simulink library "TorqueCommand"  (R2024a)
settings: Solver=VariableStepAuto  StartTime=0.0  StopTime=10.0  RelTol=1e-3
values from neighbouring files (symbols this model uses):
  RegenEnable : value not decoded    [TorqueCommand.sldd]
  TCEnable : value not decoded    [TorqueCommand.sldd]
undefined symbols (not defined in the file or in its folder): raptor_xcp_function
libraries: Raptor_lib x37, Utilities x7, simulink x6, slpidlib x1
settings Model: Creator=serga  LastModifiedBy=hyuga
settings ConfigComp: CovBoundaryAbsTol=1.0e-5

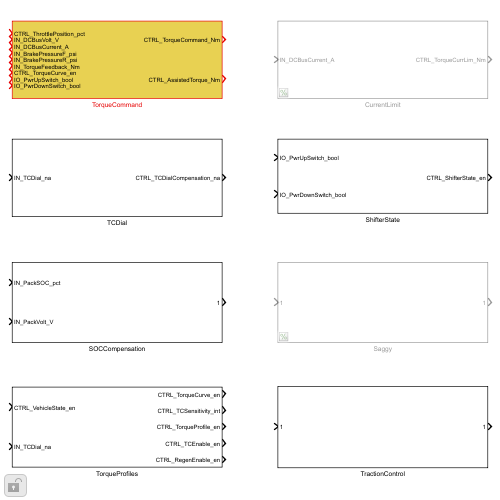
[thumbnail: Simulink's stored preview of the top-level diagram]
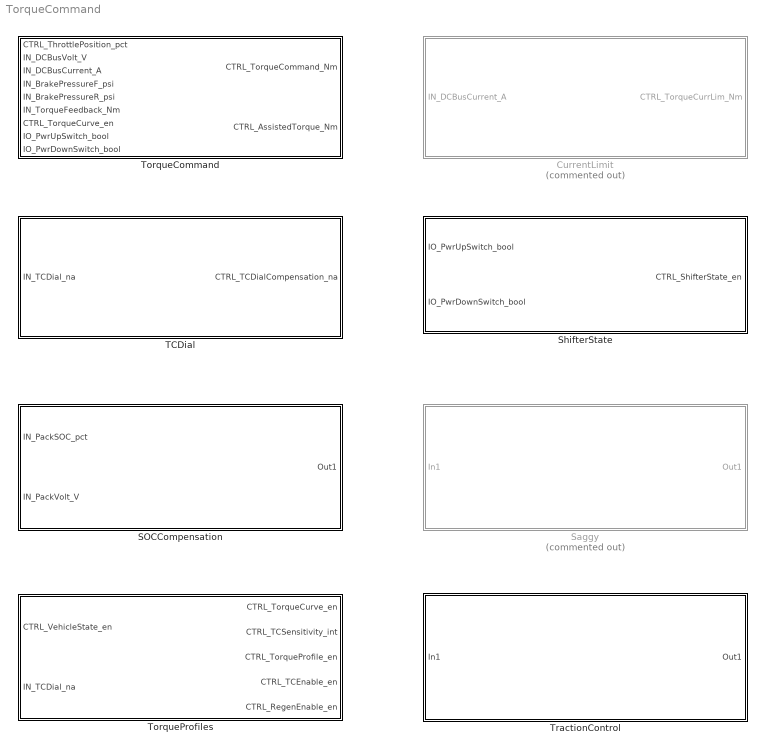
== system TorqueCommand ==
  CurrentLimit : Subsystem  Commented=on
  SOCCompensation : Subsystem
  Saggy : Subsystem  Commented=on
  ShifterState : Subsystem
  TCDial : Subsystem
  TorqueCommand : Subsystem
  TorqueProfiles : Subsystem
  TractionControl : Subsystem

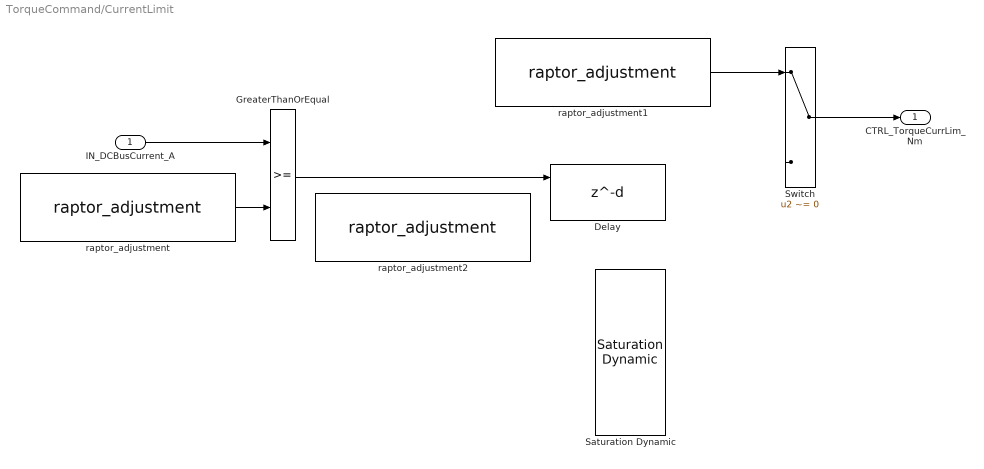
== system TorqueCommand/CurrentLimit ==
  IN_DCBusCurrent_A : Inport
  Delay : Delay  DelayLengthSource=Input port
      settings: InputPortMap=u0,p1
  GreaterThanOrEqual : RelationalOperator  OutDataTypeStr=boolean  RndMeth=Simplest  InputSameDT=off
  Saturation Dynamic : simulink/Discontinuities/Saturation Dynamic  OutMin=[]  OutMax=[]  OutDataTypeStr=Inherit: Same as second input  OutDataType=fixdt(1, 16)  OutScaling=2^-10  DoSatur=off
  Switch : Switch  Criteria=u2 ~= 0  SaturateOnIntegerOverflow=off  InputSameDT=off
  raptor_adjustment : Raptor_lib/Data Storage/raptor_adjustment  paramName='CTRL_DCBusOverCurrThresh_A'  nameSource=Parameter  initValue=125  dataType=uint8  storage=Calibration  calDispType=Number  calEnum={'False', 'True'}  calGain=1.0  calOffset=0.0  calMax=inf  calMin=-inf  calFormat='-1'  calUnit=''  calHelp=''  calAccess=1  calFunction=raptor_xcp_function(gcb)  calDispHeaders=off  calColHeaders={'Col1' 'Col2' 'Col3'}  calRowHeaders={'Row1' 'Row2' 'Row3'}
      settings: SourceProductName=Raptor
  raptor_adjustment1 : Raptor_lib/Data Storage/raptor_adjustment  paramName='CTRL_TorqueCurrLim_Nm'  nameSource=Parameter  initValue=100  dataType=double  storage=Calibration  calDispType=Number  calEnum={'False', 'True'}  calGain=1.0  calOffset=0.0  calMax=inf  calMin=-inf  calFormat='-1'  calUnit=''  calHelp=''  calAccess=1  calFunction=raptor_xcp_function(gcb)  calDispHeaders=off  calColHeaders={'Col1' 'Col2' 'Col3'}  calRowHeaders={'Row1' 'Row2' 'Row3'}
      settings: SourceProductName=Raptor
  raptor_adjustment2 : Raptor_lib/Data Storage/raptor_adjustment  paramName='CTRL_TorqueCurrLim_Nm'  nameSource=Parameter  initValue=100  dataType=double  storage=Calibration  calDispType=Number  calEnum={'False', 'True'}  calGain=1.0  calOffset=0.0  calMax=inf  calMin=-inf  calFormat='-1'  calUnit=''  calHelp=''  calAccess=1  calFunction=raptor_xcp_function(gcb)  calDispHeaders=off  calColHeaders={'Col1' 'Col2' 'Col3'}  calRowHeaders={'Row1' 'Row2' 'Row3'}
      settings: SourceProductName=Raptor
  CTRL_TorqueCurrLim_Nm : Outport
  wires:
  IN_DCBusCurrent_A/1 -> GreaterThanOrEqual/1
  raptor_adjustment/1 -> GreaterThanOrEqual/2
  GreaterThanOrEqual/1 -> Delay/1
  Switch/1 -> CTRL_TorqueCurrLim_Nm/1
  raptor_adjustment1/1 -> Switch/1

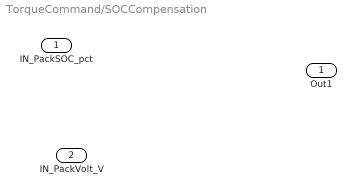
== system TorqueCommand/SOCCompensation ==
  IN_PackSOC_pct : Inport
  IN_PackVolt_V : Inport  Port=2
  Out1 : Outport

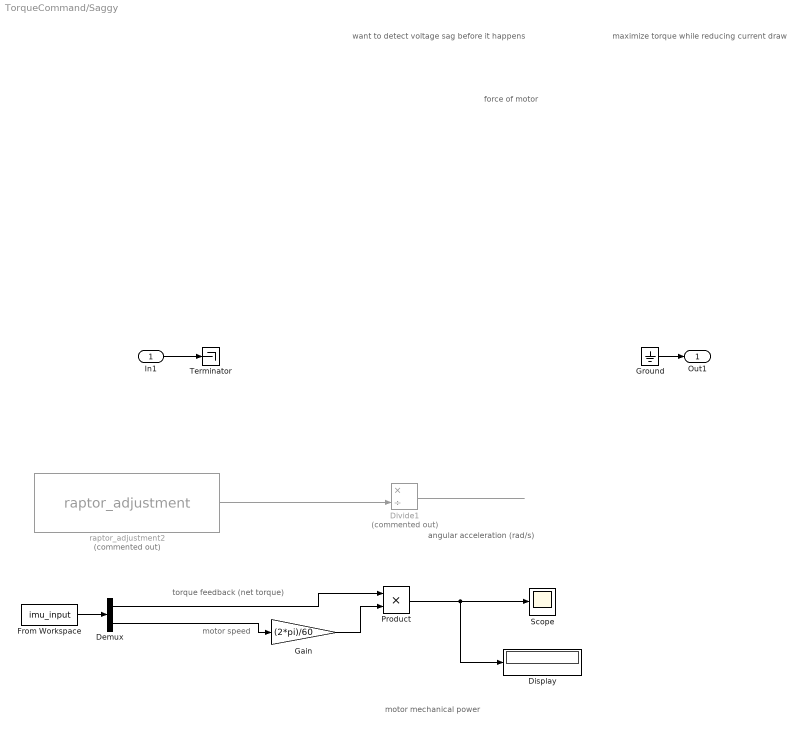
== system TorqueCommand/Saggy ==
  note: motor speed
  note: angular acceleration (rad/s)
  note: torque feedback (net torque)
  note: force of motor
  note: want to detect voltage sag before it happens
  note: maximize torque while reducing current draw
  note: motor mechanical power
  In1 : Inport
  Demux : Demux  Outputs=2
  Display : Display
  Divide1 : Product  Commented=on  Inputs=*/
  From Workspace : FromWorkspace  VariableName=imu_input  SampleTime=-1
  Gain : Gain  Gain=(2*pi)/60
  Ground : Ground
  Product : Product
  Scope : Scope
  Terminator : Terminator
  raptor_adjustment2 : Raptor_lib/Data Storage/raptor_adjustment  Commented=on  paramName='CTRL_MotorIntertia_kgm2'  nameSource=Parameter  initValue=0.0383  dataType=double  storage=Calibration  calDispType=Number  calEnum={'False', 'True'}  calGain=1.0  calOffset=0.0  calMax=inf  calMin=-inf  calFormat='-1'  calUnit=''  calHelp=''  calAccess=1  calFunction=raptor_xcp_function(gcb)  calDispHeaders=off  calColHeaders={'Col1' 'Col2' 'Col3'}  calRowHeaders={'Row1' 'Row2' 'Row3'}
      settings: SourceProductName=Raptor
  Out1 : Outport
  wires:
  In1/1 -> Terminator/1
  Ground/1 -> Out1/1
  raptor_adjustment2/1 -> Divide1/2
  Divide1/1 -> ?
  Gain/1 -> Product/2
  From Workspace/1 -> Demux/1
  Demux/1 -> Product/1
  Demux/2 -> Gain/1
  Product/1 -> Display/1, Scope/1

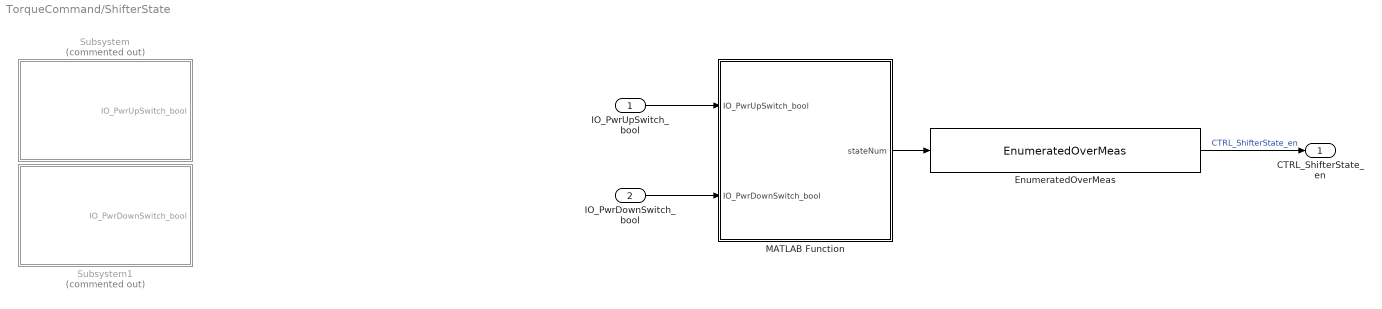
== system TorqueCommand/ShifterState ==
  IO_PwrUpSwitch_bool : Inport
  IO_PwrDownSwitch_bool : Inport  Port=2
  EnumeratedOverMeas : Utilities/EnumeratedOverMeas  sigName='CTRL_ShifterState_en'  enumName='TorqueState'
  MATLAB Function : MATLAB Function  TreatAsAtomicUnit=on
  Subsystem : Subsystem  Commented=on
  Subsystem1 : Subsystem  Commented=on
  CTRL_ShifterState_en : Outport
  wires:
  EnumeratedOverMeas/1 -> CTRL_ShifterState_en/1  "CTRL_ShifterState_en"
  MATLAB Function/1(stateNum) -> EnumeratedOverMeas/1
  IO_PwrDownSwitch_bool/1 -> MATLAB Function/2(IO_PwrDownSwitch_bool)
  IO_PwrUpSwitch_bool/1 -> MATLAB Function/1(IO_PwrUpSwitch_bool)

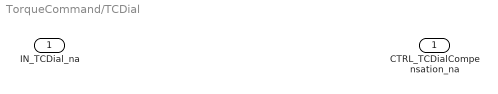
== system TorqueCommand/TCDial ==
  IN_TCDial_na : Inport
  CTRL_TCDialCompensation_na : Outport

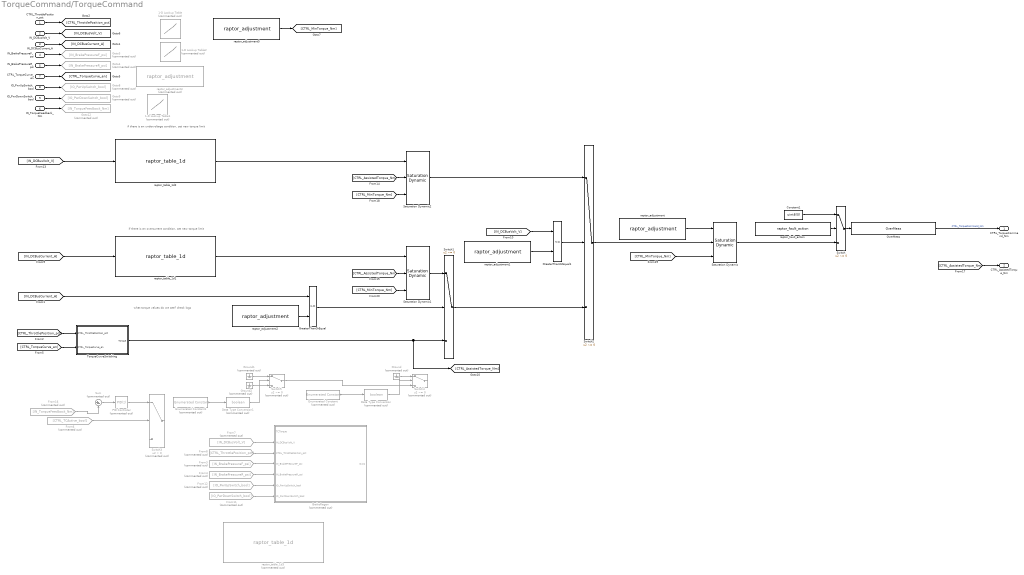
== system TorqueCommand/TorqueCommand ==
  note: if there is an undervoltage condition, set new torque limit
  note: what torque values do we see? check logs
  note: if there is an overcurrent condition, set new torque limit
  CTRL_ThrottlePosition_pct : Inport
  IN_DCBusVolt_V : Inport  Port=2
  IN_DCBusCurrent_A : Inport  Port=3
  IN_BrakePressureF_psi : Inport  Port=4
  IN_BrakePressureR_psi : Inport  Port=5
  IN_TorqueFeedback_Nm : Inport  Port=6
  CTRL_TorqueCurve_en : Inport  Port=7
  IO_PwrUpSwitch_bool : Inport  Port=8
  IO_PwrDownSwitch_bool : Inport  Port=9
  1-D Lookup Table : Lookup_n-D  Commented=on  NumberOfTableDimensions=1  BreakpointsForDimension1=[0;50;100;120;130;140;150;160;170;180;190;200;205;210;215;220;225;230;235;240;245;250;255;260;265;270;275;280;285;290;295;300]  Table=[200;200;200;200;200;200;200;200;200;200;200;200;200;200;200;200;200;200;200;200;200;200;195;190;185;180;175;170;165;160;155;150]  InternalRulePriority=Speed  RndMeth=Simplest
  1-D Lookup Table1 : Lookup_n-D  Commented=on  NumberOfTableDimensions=1  BreakpointsForDimension1=[0;5;10;15;20;25;30;35;40;45;50;55;60;65;70;75;80;85;90;95;100]  Table=[0;3;6;9;12;15;25;35;45;55;65;75;85;95;105;115;135;155;175;195;200]  InternalRulePriority=Speed  RndMeth=Simplest
  1-D Lookup Table2 : Lookup_n-D  Commented=on  NumberOfTableDimensions=1  BreakpointsForDimension1=[0;100;200;205;210;215;220;225;230;235;240;245;250;255;260;265;270;275;280;285;290;300;310;320;330;400]  Table=[0;0;0;25;50;100;125;150;155;160;165;170;175;180;185;190;192;194;196;198;200;200;200;200;200;200]  InternalRulePriority=Speed  RndMeth=Simplest
  BrakeRegen : Subsystem  Commented=on
  Constant1 : Constant  Value=uint8(0)
  Data Type Conversion : DataTypeConversion  Commented=on  OutDataTypeStr=boolean  SaturateOnIntegerOverflow=off  RndMeth=Floor
  Data Type Conversion1 : DataTypeConversion  Commented=on  OutDataTypeStr=boolean  SaturateOnIntegerOverflow=off  RndMeth=Floor
  Enumerated Constant : simulink/Sources/Enumerated Constant  Commented=on  OutDataTypeStr=Enum: RegenEnable  Value=RegenEnable.On  SampleTime=inf
  Enumerated Constant1 : simulink/Sources/Enumerated Constant  Commented=on  OutDataTypeStr=Enum: TCEnable  Value=TCEnable.On  SampleTime=inf
  From11 : From  Commented=on  GotoTag=IO_PwrDownSwitch_bool
  From12 : From  Commented=on  GotoTag=IO_PwrUpSwitch_bool
  From16 : From  Commented=on  GotoTag=IN_TorqueFeedback_Nm
  From3 : From  Commented=on  GotoTag=IN_BrakePressureF_psi
  From4 : From  Commented=on  GotoTag=IN_BrakePressureR_psi
  From6 : From  Commented=on  GotoTag=CTRL_TCActive_bool
  From7 : From  Commented=on  GotoTag=IN_DCBusVolt_V
  From8 : From  Commented=on  GotoTag=CTRL_ThrottlePosition_pct
  Goto12 : Goto  Commented=on  GotoTag=IN_TorqueFeedback_Nm
  Goto3 : Goto  Commented=on  GotoTag=IN_BrakePressureF_psi
  Goto4 : Goto  Commented=on  GotoTag=IN_BrakePressureR_psi
  Goto8 : Goto  Commented=on  GotoTag=IO_PwrUpSwitch_bool
  Goto9 : Goto  Commented=on  GotoTag=IO_PwrDownSwitch_bool
  GreaterThanOrEqual : RelationalOperator  OutDataTypeStr=boolean  RndMeth=Simplest  InputSameDT=off
  GreaterThanOrEqual1 : RelationalOperator  Operator=<=  OutDataTypeStr=boolean  RndMeth=Simplest  InputSameDT=off
  Ground : Ground  Commented=on
  Ground1 : Ground  Commented=on
  Ground2 : Ground  Commented=on
  OverMeas : Utilities/OverMeas  sigName='CTRL_TorqueCommand_Nm'  minimum=0  maximum=240
  PID Controller : slpidlib/PID Controller  Commented=on  Controller=PID  Form=Parallel  TimeDomain=Discrete-time  UseExternalTs=off  SampleTime=-1  IntegratorMethod=Forward Euler  FilterMethod=Forward Euler  ControllerParametersSource=internal  P=1  I=1  UseKiTs=off  D=0  UseExternalDerivativeSource=off  N=100  UseFilter=on  TunerSelectOption=Transfer Function Based (PID Tuner App)  InitialConditionSource=internal  InitialConditionForIntegrator=0  InitialConditionForFilter=0  DifferentiatorICPrevScaledInput=0  ExternalReset=none  TrackingMode=off  Kt=1  LimitOutput=off  SatLimitsSource=internal  UpperSaturationLimit=inf  LowerSaturationLimit=-inf  LinearizeAsGain=on  AntiWindupMode=none  Kb=1  LimitIntegrator=off  UpperIntegratorSaturationLimit=inf  LowerIntegratorSaturationLimit=-inf  POutMin=[]  POutMax=[]  IOutMin=[]  IOutMax=[]  DOutMin=[]  DOutMax=[]  NOutMin=[]  NOutMax=[]  SumOutMin=[]  SumOutMax=[]  SaturationOutMin=[]  SaturationOutMax=[]  PParamMin=[]  PParamMax=[]  IParamMin=[]  IParamMax=[]  DParamMin=[]  DParamMax=[]  NParamMin=[]  NParamMax=[]  KbParamMin=[]  KbParamMax=[]  KtParamMin=[]  KtParamMax=[]  KbOutMin=[]  KbOutMax=[]  KtOutMin=[]  KtOutMax=[]  IntegratorOutMin=[]  IntegratorOutMax=[]  FilterOutMin=[]  FilterOutMax=[]  SumI1OutMin=[]  SumI1OutMax=[]  SumI2OutMin=[]  SumI2OutMax=[]  SumI3OutMin=[]  SumI3OutMax=[]  SumI4OutMin=[]  SumI4OutMax=[]  SumDOutMin=[]  SumDOutMax=[]  DifferentiatorOutMin=[]  DifferentiatorOutMax=[]  FilterDiffOutCoefMin=[]  FilterDiffOutCoefMax=[]  ReciprocalOutMin=[]  ReciprocalOutMax=[]  SumDenOutMin=[]  SumDenOutMax=[]  SumNumOutMin=[]  SumNumOutMax=[]  DivideOutMin=[]  DivideOutMax=[]  UdiffTsProdOutMin=[]  UdiffTsProdOutMax=[]  NTsProdOutMin=[]  NTsProdOutMax=[]  UintegralTsProdOutMin=[]  UintegralTsProdOutMax=[]  UngainTsProdOutMin=[]  UngainTsProdOutMax=[]  ClampingZeroOutDataTypeStr=Inherit: Inherit via back propagation  ClampingZeroOutMin=[]  ClampingZeroOutMax=[]  FilterDenConstantOutDataTypeStr=Inherit: Inherit via back propagation  FilterDenConstantOutMin=[]  FilterDenConstantOutMax=[]  PCopyOutDataTypeStr=Inherit: Inherit via back propagation  PCopyOutMin=[]  PCopyOutMax=[]  NCopyOutDataTypeStr=Inherit: Inherit via back propagation  NCopyOutMin=[]  NCopyOutMax=[]  IntegratorContinuousStateAttributes=''  IntegratorStateMustResolveToSignalObject=off  IntegratorRTWStateStorageClass=Auto  FilterContinuousStateAttributes=''  FilterStateMustResolveToSignalObject=off  FilterRTWStateStorageClass=Auto  ParallelPVariant=InternalParameters  IdealPVariant=Disabled  IVariant=InternalParameters  DVariant=InternalParameters  IntegratorVariant=Discrete  SatVariant=Disabled  AWVariant=Passthrough  PCopyVariant=Disabled  TRVariant=Disabled  FdbkBlocksVariant=Forward  IdealPFdbkVariant=Disabled  SatFdbkVariant=Disabled  DerivativeFilterVariant=ForwardEulerFilter  NVariant=InternalParameters  NCopyVariant=Disabled  FilterICVariant=InternalICsFilter  IntegratorICVariant=InternalICs  ExternalResetVariant=Disabled  TRSumVariant=Passthrough  SumFdbkVariant=Disabled  SumVariant=Sum_PID  TsampFilterVariant=InternalTs  TsampNgainVariant=Passthrough  TsampIntegralVariant=Disabled_SignalSpec  ExternalSaturationOutDataTypeStr=Inherit: Same as second input  DerivativeSourceVariant=ErrorSignal
  Saturation Dynamic : simulink/Discontinuities/Saturation Dynamic  OutMin=[]  OutMax=[]  OutDataTypeStr=Inherit: Same as second input  OutDataType=fixdt(1, 16)  OutScaling=2^-10  DoSatur=off
  Saturation Dynamic1 : simulink/Discontinuities/Saturation Dynamic  OutMin=[]  OutMax=[]  OutDataTypeStr=Inherit: Same as second input  OutDataType=fixdt(1, 16)  OutScaling=2^-10  DoSatur=off
  Saturation Dynamic2 : simulink/Discontinuities/Saturation Dynamic  OutMin=[]  OutMax=[]  OutDataTypeStr=Inherit: Same as second input  OutDataType=fixdt(1, 16)  OutScaling=2^-10  DoSatur=off
  Sum : Sum  Commented=on  Inputs=|+-
  Switch : Switch  Criteria=u2 ~= 0  SaturateOnIntegerOverflow=off  InputSameDT=off
  Switch1 : Switch  Criteria=u2 ~= 0  SaturateOnIntegerOverflow=off  InputSameDT=off
  Switch2 : Switch  Criteria=u2 ~= 0  OutDataTypeStr=single  SaturateOnIntegerOverflow=off  InputSameDT=off
  Switch3 : Switch  Commented=on  Criteria=u2 > Threshold  SaturateOnIntegerOverflow=off  InputSameDT=off
  Switch4 : Switch  Commented=on  Criteria=u2 ~= 0  SaturateOnIntegerOverflow=off  InputSameDT=off
  Switch5 : Switch  Commented=on  Criteria=u2 ~= 0  SaturateOnIntegerOverflow=off  InputSameDT=off
  TorqueCurveSwitching : Subsystem
  raptor_adjustment : Raptor_lib/Data Storage/raptor_adjustment  paramName='CTRL_MaxTorque'  nameSource=Parameter  initValue=230  dataType=single  storage=Calibration  calDispType=Number  calEnum={'False', 'True'}  calGain=1.0  calOffset=0.0  calMax=250  calMin=0  calFormat='-1'  calUnit=''  calHelp=''  calAccess=1  calFunction=raptor_xcp_function(gcb)  calDispHeaders=off  calColHeaders={'Col1' 'Col2' 'Col3'}  calRowHeaders={'Row1' 'Row2' 'Row3'}
      settings: SourceProductName=Raptor
  raptor_adjustment1 : Raptor_lib/Data Storage/raptor_adjustment  paramName='CTRL_DCBusUnderVoltThresh_V'  nameSource=Parameter  initValue=250  dataType=single  storage=Calibration  calDispType=Number  calEnum={'False', 'True'}  calGain=1.0  calOffset=0.0  calMax=240  calMin=-inf  calFormat='-1'  calUnit=''  calHelp=''  calAccess=1  calFunction=raptor_xcp_function(gcb)  calDispHeaders=off  calColHeaders={'Col1' 'Col2' 'Col3'}  calRowHeaders={'Row1' 'Row2' 'Row3'}
      settings: SourceProductName=Raptor
  raptor_adjustment2 : Raptor_lib/Data Storage/raptor_adjustment  paramName='CTRL_DCBusOverCurrThresh_A'  nameSource=Parameter  initValue=125  dataType=single  storage=Calibration  calDispType=Number  calEnum={'False', 'True'}  calGain=1.0  calOffset=0.0  calMax=240  calMin=-inf  calFormat='-1'  calUnit=''  calHelp=''  calAccess=1  calFunction=raptor_xcp_function(gcb)  calDispHeaders=off  calColHeaders={'Col1' 'Col2' 'Col3'}  calRowHeaders={'Row1' 'Row2' 'Row3'}
      settings: SourceProductName=Raptor
  raptor_adjustment3 : Raptor_lib/Data Storage/raptor_adjustment  Commented=on  paramName='CTRL_TorqueCurrLim_Nm'  nameSource=Parameter  initValue=100  dataType=single  storage=Calibration  calDispType=Number  calEnum={'False', 'True'}  calGain=1.0  calOffset=0.0  calMax=inf  calMin=-inf  calFormat='-1'  calUnit=''  calHelp=''  calAccess=1  calFunction=raptor_xcp_function(gcb)  calDispHeaders=off  calColHeaders={'Col1' 'Col2' 'Col3'}  calRowHeaders={'Row1' 'Row2' 'Row3'}
      settings: SourceProductName=Raptor
  raptor_adjustment5 : Raptor_lib/Data Storage/raptor_adjustment  paramName='CTRL_MinTorque'  nameSource=Parameter  initValue=-230  dataType=single  storage=Calibration  calDispType=Number  calEnum={'False', 'True'}  calGain=1.0  calOffset=0.0  calMax=230  calMin=-250  calFormat='-1'  calUnit=''  calHelp=''  calAccess=1  calFunction=raptor_xcp_function(gcb)  calDispHeaders=off  calColHeaders={'Col1' 'Col2' 'Col3'}  calRowHeaders={'Row1' 'Row2' 'Row3'}
      settings: SourceProductName=Raptor
  raptor_fault_action : Raptor_lib/Faults/raptor_fault_action  actionName='TorqueCmdOverride'  calVisible=on  calAccess=1  calFunction='System | FaultManager | FaultAction'
      settings: SourceProductName=Raptor
  raptor_table_1d1 : Raptor_lib/Table Lookup/raptor_table_1d  dataName='CTRL_CurrentToLimTorqueCmd_1D'  initValue=[200;200;200;200;200;200;200;200;200;200;200;200;200;200;200;200;200;200;200;200;200;200;195;190;185;180;175;170;165;160;155;150]  dataType=single  storage=Calibration  initValueX=[0;50;100;120;130;140;150;160;170;180;190;200;205;210;215;220;225;230;235;240;245;250;255;260;265;270;275;280;285;290;295;300]  dataTypeXY=single  storageXY=Calibration  calVisible=on  showTable=on  calGain=1.0  calOffset=0.0  calMax=Inf  calMin=-Inf  calFormat='-1'  calUnit='Nm'  calHelp=''  showBreakpoint=on  dataNameX=[]  calGainX=1.0  calOffsetX=0.0  calMaxX=Inf  calMinX=-Inf  calFormatX='-1'  calUnitX='A'  calHelpX=''  calAccess=1  calFunction=raptor_xcp_function(gcb)  measureEnable=off  mName=['Data1D_Output']
      settings: SourceProductName=Raptor
  raptor_table_1d2 : Raptor_lib/Table Lookup/raptor_table_1d  dataName='CTRL_VoltageToLimTorqueCmd_1D'  initValue=[0;0;0;25;50;100;125;150;155;160;165;170;175;180;185;190;192;194;196;198;200;200;200;200;200;200]  dataType=double  storage=Calibration  initValueX=[0;100;200;205;210;215;220;225;230;235;240;245;250;255;260;265;270;275;280;285;290;300;310;320;330;400]  dataTypeXY=double  storageXY=Calibration  calVisible=on  showTable=on  calGain=1.0  calOffset=0.0  calMax=Inf  calMin=-Inf  calFormat='-1'  calUnit='Nm'  calHelp=''  showBreakpoint=on  dataNameX=[]  calGainX=1.0  calOffsetX=0.0  calMaxX=Inf  calMinX=-Inf  calFormatX='-1'  calUnitX='V'  calHelpX=''  calAccess=1  calFunction=raptor_xcp_function(gcb)  measureEnable=off  mName=['Data1D_Output']
      settings: SourceProductName=Raptor
  raptor_table_1d3 : Raptor_lib/Table Lookup/raptor_table_1d  Commented=on  dataName='CTRL_TargetSlipRatio_1D'  initValue=[0;764;1528;2293;3057;3822;4586;5350;6114;6880;7643]  dataType=single  storage=Calibration  initValueX=[12;12;12;12;12;12;11.5;11;10.5;10;8]  dataTypeXY=single  storageXY=Calibration  calVisible=on  showTable=on  calGain=1.0  calOffset=0.0  calMax=Inf  calMin=-Inf  calFormat='-1'  calUnit='pct'  calHelp=''  showBreakpoint=on  dataNameX=[]  calGainX=1.0  calOffsetX=0.0  calMaxX=Inf  calMinX=-Inf  calFormatX='-1'  calUnitX='rpm'  calHelpX=''  calAccess=1  calFunction=raptor_xcp_function(gcb)  measureEnable=off  mName=['Data1D_Output']
      settings: SourceProductName=Raptor
  CTRL_TorqueCommand_Nm : Outport
  CTRL_AssistedTorque_Nm : Outport  Port=2
  wires:
  [CTRL_MinTorque_Nm] -> Saturation Dynamic1/3
  [CTRL_MinTorque_Nm] -> Saturation Dynamic/3
  [CTRL_MinTorque_Nm] -> Saturation Dynamic2/3
  raptor_adjustment5/1 -> [CTRL_MinTorque_Nm]
  Ground2/1 -> Switch5/3
  Ground1/1 -> Switch5/1
  Data Type Conversion1/1 -> Switch5/2
  Data Type Conversion/1 -> Switch4/2
  Enumerated Constant1/1 -> Data Type Conversion1/1
  Enumerated Constant/1 -> Data Type Conversion/1
  Switch5/1 -> Switch4/3
  Ground/1 -> Switch4/1
  TorqueCurveSwitching/1(Torque) -> Switch1/3, [CTRL_AssistedTorque_Nm]
  IN_TorqueFeedback_Nm/1 -> Goto12/1
  From16/1 -> Sum/2
  PID Controller/1 -> Switch3/1
  Sum/1 -> PID Controller/1
  [CTRL_AssistedTorque_Nm] -> CTRL_AssistedTorque_Nm/1
  [CTRL_AssistedTorque_Nm] -> Saturation Dynamic1/2
  [CTRL_AssistedTorque_Nm] -> Saturation Dynamic2/2
  From11/1 -> BrakeRegen/7(IO_PwrDownSwitch_bool)
  From12/1 -> BrakeRegen/6(IO_PwrUpSwitch_bool)
  IO_PwrUpSwitch_bool/1 -> Goto8/1
  IO_PwrDownSwitch_bool/1 -> Goto9/1
  [IN_DCBusVolt_V] -> GreaterThanOrEqual1/1
  [IN_DCBusCurrent_A] -> raptor_table_1d1/1
  From8/1 -> BrakeRegen/3(CTRL_ThrottlePosition_pct)
  From7/1 -> BrakeRegen/2(IN_DCBusVolt_V)
  [CTRL_TorqueCurve_en] -> TorqueCurveSwitching/2(CTRL_TorqueCurve_en)
  CTRL_TorqueCurve_en/1 -> [CTRL_TorqueCurve_en]
  IN_BrakePressureR_psi/1 -> Goto4/1
  From4/1 -> BrakeRegen/5(IN_BrakePressureR_psi)
  IN_BrakePressureF_psi/1 -> Goto3/1
  From3/1 -> BrakeRegen/4(IN_BrakePressureF_psi)
  CTRL_ThrottlePosition_pct/1 -> [CTRL_ThrottlePosition_pct]
  IN_DCBusCurrent_A/1 -> [IN_DCBusCurrent_A]
  IN_DCBusVolt_V/1 -> [IN_DCBusVolt_V]
  [CTRL_ThrottlePosition_pct] -> TorqueCurveSwitching/1(CTRL_ThrottlePosition_pct)
  Switch2/1 -> Saturation Dynamic/2
  raptor_adjustment/1 -> Saturation Dynamic/1
  Saturation Dynamic/1 -> Switch/3
  From6/1 -> Switch3/2
  raptor_adjustment1/1 -> GreaterThanOrEqual1/2
  GreaterThanOrEqual1/1 -> Switch2/2
  Saturation Dynamic2/1 -> Switch2/1
  raptor_table_1d2/1 -> Saturation Dynamic2/1
  [IN_DCBusVolt_V] -> raptor_table_1d2/1
  raptor_table_1d1/1 -> Saturation Dynamic1/1
  Saturation Dynamic1/1 -> Switch1/1
  GreaterThanOrEqual/1 -> Switch1/2
  [IN_DCBusCurrent_A] -> GreaterThanOrEqual/1
  raptor_adjustment2/1 -> GreaterThanOrEqual/2
  Switch1/1 -> Switch2/3
  raptor_fault_action/1 -> Switch/2
  OverMeas/1 -> CTRL_TorqueCommand_Nm/1  "CTRL_TorqueCommand_Nm"
  Switch/1 -> OverMeas/1
  Constant1/1 -> Switch/1

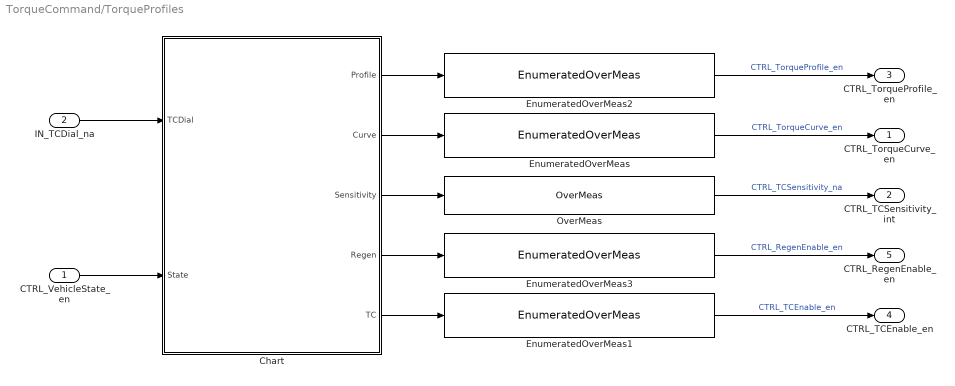
== system TorqueCommand/TorqueProfiles ==
  CTRL_VehicleState_en : Inport
  IN_TCDial_na : Inport  Port=2
  Chart : Stateflow chart  TreatAsAtomicUnit=on
  EnumeratedOverMeas : Utilities/EnumeratedOverMeas  sigName='CTRL_TorqueCurve_en'  enumName='TorqueCurve'
  EnumeratedOverMeas1 : Utilities/EnumeratedOverMeas  sigName='CTRL_TCEnable_en'  enumName='TCEnable'
  EnumeratedOverMeas2 : Utilities/EnumeratedOverMeas  sigName='CTRL_TorqueProfile_en'  enumName='TorqueProfile'
  EnumeratedOverMeas3 : Utilities/EnumeratedOverMeas  sigName='CTRL_RegenEnable_en'  enumName='RegenEnable'
  OverMeas : Utilities/OverMeas  sigName='CTRL_TCSensitivity_na'  minimum=-inf  maximum=inf
  CTRL_TorqueCurve_en : Outport
  CTRL_TCSensitivity_int : Outport  Port=2
  CTRL_TorqueProfile_en : Outport  Port=3
  CTRL_TCEnable_en : Outport  Port=4
  CTRL_RegenEnable_en : Outport  Port=5
  wires:
  EnumeratedOverMeas1/1 -> CTRL_TCEnable_en/1  "CTRL_TCEnable_en"
  EnumeratedOverMeas3/1 -> CTRL_RegenEnable_en/1  "CTRL_RegenEnable_en"
  Chart/5(TC) -> EnumeratedOverMeas1/1
  Chart/4(Regen) -> EnumeratedOverMeas3/1
  Chart/2(Curve) -> EnumeratedOverMeas/1
  Chart/1(Profile) -> EnumeratedOverMeas2/1
  CTRL_VehicleState_en/1 -> Chart/2(State)
  EnumeratedOverMeas2/1 -> CTRL_TorqueProfile_en/1  "CTRL_TorqueProfile_en"
  IN_TCDial_na/1 -> Chart/1(TCDial)
  Chart/3(Sensitivity) -> OverMeas/1
  OverMeas/1 -> CTRL_TCSensitivity_int/1  "CTRL_TCSensitivity_na"
  EnumeratedOverMeas/1 -> CTRL_TorqueCurve_en/1  "CTRL_TorqueCurve_en"

== system TorqueCommand/TractionControl ==
  In1 : Inport
  Out1 : Outport
  wires:
  In1/1 -> Out1/1

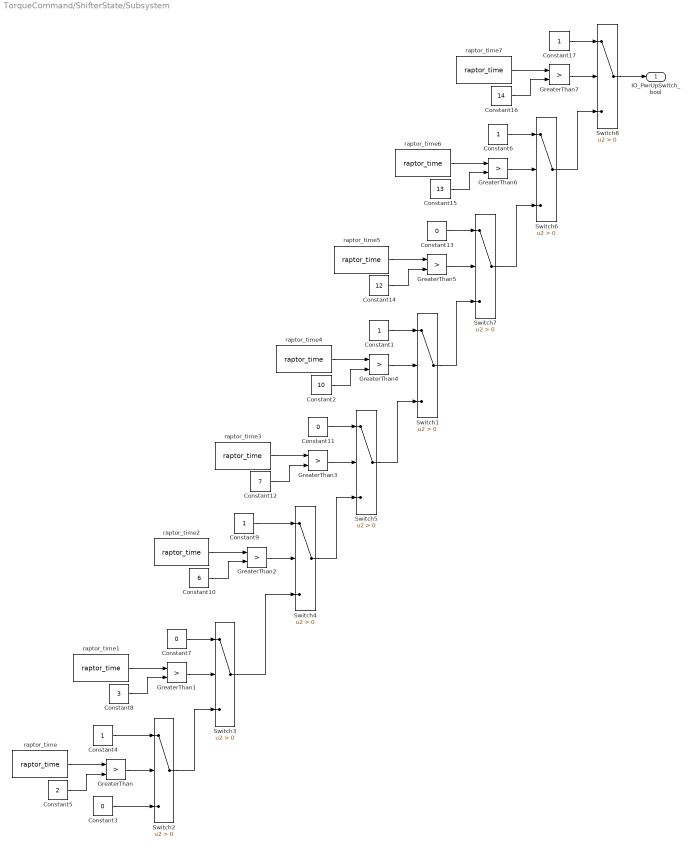
== system TorqueCommand/ShifterState/Subsystem ==
  Constant{1,4,6,9,17} (5 alike) : Constant
  Constant10 : Constant  Value=6
  Constant{3,7,11,13} (4 alike) : Constant  Value=0
  Constant12 : Constant  Value=7
  Constant14 : Constant  Value=12
  Constant15 : Constant  Value=13
  Constant16 : Constant  Value=14
  Constant2 : Constant  Value=10
  Constant5 : Constant  Value=2
  Constant8 : Constant  Value=3
  GreaterThan{,1..7} (8 alike) : RelationalOperator  Operator=>  OutDataTypeStr=boolean  RndMeth=Simplest  InputSameDT=off
  Switch{1..8} (8 alike) : Switch  Criteria=u2 > Threshold  SaturateOnIntegerOverflow=off  InputSameDT=off
  raptor_time{,1..7} (8 alike) : Raptor_lib/Triggers/raptor_time  unit=seconds
      settings: SourceProductName=Raptor
  IO_PwrUpSwitch_bool : Outport
  wires:
  Switch8/1 -> IO_PwrUpSwitch_bool/1
  GreaterThan7/1 -> Switch8/2
  Switch6/1 -> Switch8/3
  Constant16/1 -> GreaterThan7/2
  Constant17/1 -> Switch8/1
  raptor_time7/1 -> GreaterThan7/1
  Switch1/1 -> Switch7/3
  Constant14/1 -> GreaterThan5/2
  Constant15/1 -> GreaterThan6/2
  raptor_time5/1 -> GreaterThan5/1
  Constant6/1 -> Switch6/1
  GreaterThan5/1 -> Switch7/2
  GreaterThan6/1 -> Switch6/2
  raptor_time6/1 -> GreaterThan6/1
  Switch7/1 -> Switch6/3
  Constant13/1 -> Switch7/1
  Constant2/1 -> GreaterThan4/2
  Switch5/1 -> Switch1/3
  raptor_time4/1 -> GreaterThan4/1
  GreaterThan4/1 -> Switch1/2
  Constant1/1 -> Switch1/1
  Constant11/1 -> Switch5/1
  Constant8/1 -> GreaterThan1/2
  raptor_time1/1 -> GreaterThan1/1
  GreaterThan1/1 -> Switch3/2
  Switch4/1 -> Switch5/3
  GreaterThan3/1 -> Switch5/2
  raptor_time3/1 -> GreaterThan3/1
  raptor_time2/1 -> GreaterThan2/1
  Switch3/1 -> Switch4/3
  Constant10/1 -> GreaterThan2/2
  raptor_time/1 -> GreaterThan/1
  GreaterThan/1 -> Switch2/2
  Constant9/1 -> Switch4/1
  Constant5/1 -> GreaterThan/2
  Constant7/1 -> Switch3/1
  Constant3/1 -> Switch2/3
  Constant4/1 -> Switch2/1
  Switch2/1 -> Switch3/3
  Constant12/1 -> GreaterThan3/2
  GreaterThan2/1 -> Switch4/2

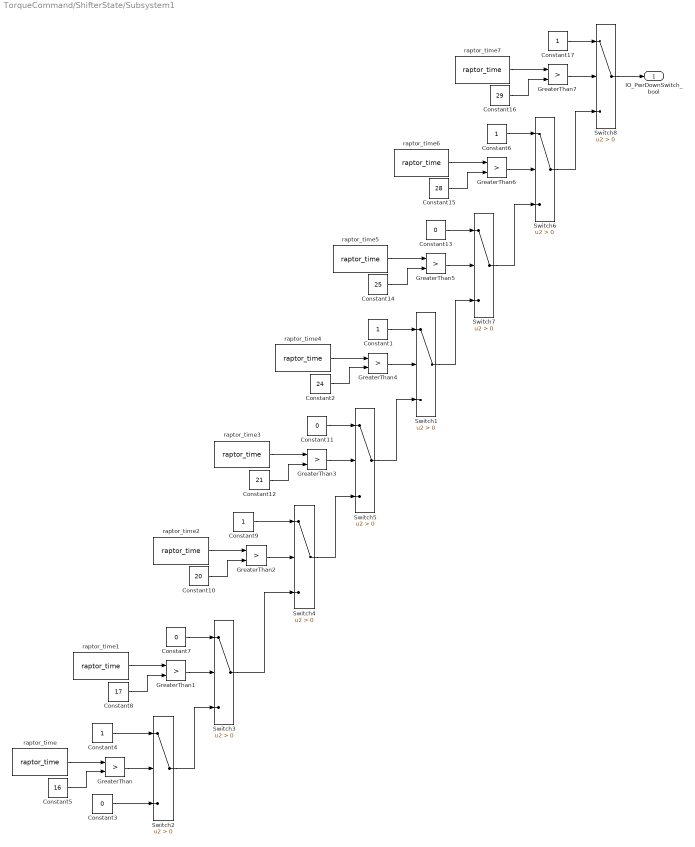
== system TorqueCommand/ShifterState/Subsystem1 ==
  Constant{1,4,6,9,17} (5 alike) : Constant
  Constant10 : Constant  Value=20
  Constant{3,7,11,13} (4 alike) : Constant  Value=0
  Constant12 : Constant  Value=21
  Constant14 : Constant  Value=25
  Constant15 : Constant  Value=28
  Constant16 : Constant  Value=29
  Constant2 : Constant  Value=24
  Constant5 : Constant  Value=16
  Constant8 : Constant  Value=17
  GreaterThan{,1..7} (8 alike) : RelationalOperator  Operator=>  OutDataTypeStr=boolean  RndMeth=Simplest  InputSameDT=off
  Switch{1..8} (8 alike) : Switch  Criteria=u2 > Threshold  SaturateOnIntegerOverflow=off  InputSameDT=off
  raptor_time{,1..7} (8 alike) : Raptor_lib/Triggers/raptor_time  unit=seconds
      settings: SourceProductName=Raptor
  IO_PwrDownSwitch_bool : Outport
  wires:
  Switch8/1 -> IO_PwrDownSwitch_bool/1
  GreaterThan7/1 -> Switch8/2
  Switch6/1 -> Switch8/3
  Constant16/1 -> GreaterThan7/2
  Constant17/1 -> Switch8/1
  raptor_time7/1 -> GreaterThan7/1
  Switch1/1 -> Switch7/3
  Constant14/1 -> GreaterThan5/2
  Constant15/1 -> GreaterThan6/2
  raptor_time5/1 -> GreaterThan5/1
  Constant6/1 -> Switch6/1
  GreaterThan5/1 -> Switch7/2
  GreaterThan6/1 -> Switch6/2
  raptor_time6/1 -> GreaterThan6/1
  Switch7/1 -> Switch6/3
  Constant13/1 -> Switch7/1
  Constant2/1 -> GreaterThan4/2
  Switch5/1 -> Switch1/3
  raptor_time4/1 -> GreaterThan4/1
  GreaterThan4/1 -> Switch1/2
  Constant1/1 -> Switch1/1
  Constant11/1 -> Switch5/1
  Constant8/1 -> GreaterThan1/2
  raptor_time1/1 -> GreaterThan1/1
  GreaterThan1/1 -> Switch3/2
  Switch4/1 -> Switch5/3
  GreaterThan3/1 -> Switch5/2
  raptor_time3/1 -> GreaterThan3/1
  raptor_time2/1 -> GreaterThan2/1
  Switch3/1 -> Switch4/3
  Constant10/1 -> GreaterThan2/2
  raptor_time/1 -> GreaterThan/1
  GreaterThan/1 -> Switch2/2
  Constant9/1 -> Switch4/1
  Constant5/1 -> GreaterThan/2
  Constant7/1 -> Switch3/1
  Constant3/1 -> Switch2/3
  Constant4/1 -> Switch2/1
  Switch2/1 -> Switch3/3
  Constant12/1 -> GreaterThan3/2
  GreaterThan2/1 -> Switch4/2

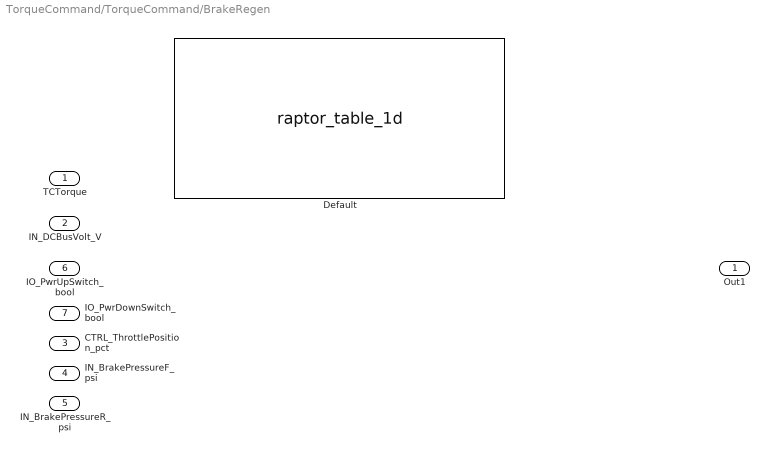
== system TorqueCommand/TorqueCommand/BrakeRegen ==
  TCTorque : Inport
  IN_DCBusVolt_V : Inport  Port=2
  CTRL_ThrottlePosition_pct : Inport  Port=3
  IN_BrakePressureF_psi : Inport  Port=4
  IN_BrakePressureR_psi : Inport  Port=5
  IO_PwrUpSwitch_bool : Inport  Port=6
  IO_PwrDownSwitch_bool : Inport  Port=7
  Default : Raptor_lib/Table Lookup/raptor_table_1d  dataName='CTRL_ThrottleToTorqueCmd_1D'  initValue=[0;3;6;9;12;15;25;35;45;55;65;75;85;95;105;115;135;155;175;195;200]  dataType=single  storage=Calibration  initValueX=[0;5;10;15;20;25;30;35;40;45;50;55;60;65;70;75;80;85;90;95;100]  dataTypeXY=single  storageXY=Calibration  calVisible=on  showTable=on  calGain=1.0  calOffset=0.0  calMax=Inf  calMin=-Inf  calFormat='-1'  calUnit='pct'  calHelp=''  showBreakpoint=on  dataNameX=[]  calGainX=1.0  calOffsetX=0.0  calMaxX=Inf  calMinX=-Inf  calFormatX='-1'  calUnitX='Nm'  calHelpX=''  calAccess=1  calFunction=raptor_xcp_function(gcb)  measureEnable=off  mName=['Data1D_Output']
      settings: SourceProductName=Raptor
  Out1 : Outport

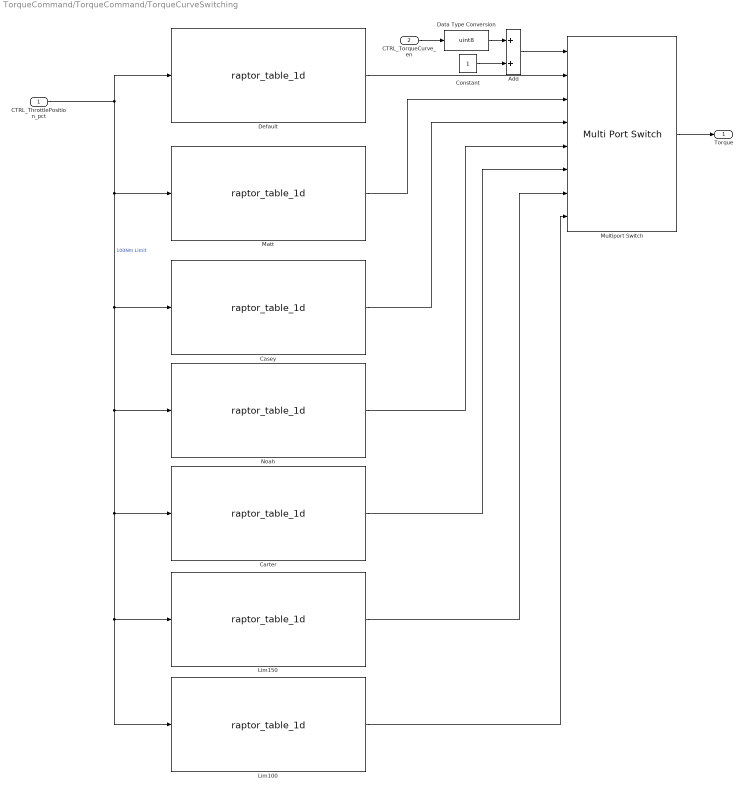
== system TorqueCommand/TorqueCommand/TorqueCurveSwitching ==
  CTRL_ThrottlePosition_pct : Inport
  CTRL_TorqueCurve_en : Inport  Port=2
  Add : Sum
  Carter : Raptor_lib/Table Lookup/raptor_table_1d  dataName='CTRL_ThrottleToTorqueCmdCarter_1D'  initValue=[0;1;3;6;11;18;25;34;45;57;70;85;101;118;137;158;179;202;227;230;230]  dataType=single  storage=Calibration  initValueX=[0;5;10;15;20;25;30;35;40;45;50;55;60;65;70;75;80;85;90;95;100]  dataTypeXY=single  storageXY=Calibration  calVisible=on  showTable=on  calGain=1.0  calOffset=0.0  calMax=Inf  calMin=-Inf  calFormat='-1'  calUnit='pct'  calHelp=''  showBreakpoint=on  dataNameX=[]  calGainX=1.0  calOffsetX=0.0  calMaxX=Inf  calMinX=-Inf  calFormatX='-1'  calUnitX='Nm'  calHelpX=''  calAccess=1  calFunction=raptor_xcp_function(gcb)  measureEnable=off  mName=['Data1D_Output']
      settings: SourceProductName=Raptor
  Casey : Raptor_lib/Table Lookup/raptor_table_1d  dataName='CTRL_ThrottleToTorqueCmdCasey_1D'  initValue=[0;3;6;9;12;15;25;35;45;55;65;75;85;95;105;115;135;155;175;195;200]  dataType=single  storage=Calibration  initValueX=[0;5;10;15;20;25;30;35;40;45;50;55;60;65;70;75;80;85;90;95;100]  dataTypeXY=single  storageXY=Calibration  calVisible=on  showTable=on  calGain=1.0  calOffset=0.0  calMax=Inf  calMin=-Inf  calFormat='-1'  calUnit='pct'  calHelp=''  showBreakpoint=on  dataNameX=[]  calGainX=1.0  calOffsetX=0.0  calMaxX=Inf  calMinX=-Inf  calFormatX='-1'  calUnitX='Nm'  calHelpX=''  calAccess=1  calFunction=raptor_xcp_function(gcb)  measureEnable=off  mName=['Data1D_Output']
      settings: SourceProductName=Raptor
  Constant : Constant
  Data Type Conversion : DataTypeConversion  OutDataTypeStr=uint8  SaturateOnIntegerOverflow=off  RndMeth=Floor
  Default : Raptor_lib/Table Lookup/raptor_table_1d  dataName='CTRL_ThrottleToTorqueCmdDef_1D'  initValue=[0;3;6;9;12;15;25;35;45;55;65;75;85;95;105;115;135;155;175;195;200]  dataType=single  storage=Calibration  initValueX=[0;5;10;15;20;25;30;35;40;45;50;55;60;65;70;75;80;85;90;95;100]  dataTypeXY=single  storageXY=Calibration  calVisible=on  showTable=on  calGain=1.0  calOffset=0.0  calMax=Inf  calMin=-Inf  calFormat='-1'  calUnit='pct'  calHelp=''  showBreakpoint=on  dataNameX=[]  calGainX=1.0  calOffsetX=0.0  calMaxX=Inf  calMinX=-Inf  calFormatX='-1'  calUnitX='Nm'  calHelpX=''  calAccess=1  calFunction=raptor_xcp_function(gcb)  measureEnable=off  mName=['Data1D_Output']
      settings: SourceProductName=Raptor
  Lim100 : Raptor_lib/Table Lookup/raptor_table_1d  dataName='CTRL_ThrottleToTorqueCmd100_1D'  initValue=[0;8;17;25;33;40;48;55;62;68;74;79;84;88;92;95;97;99;100;100;100]  dataType=single  storage=Calibration  initValueX=[0;5;10;15;20;25;30;35;40;45;50;55;60;65;70;75;80;85;90;95;100]  dataTypeXY=single  storageXY=Calibration  calVisible=on  showTable=on  calGain=1.0  calOffset=0.0  calMax=Inf  calMin=-Inf  calFormat='-1'  calUnit='pct'  calHelp=''  showBreakpoint=on  dataNameX=[]  calGainX=1.0  calOffsetX=0.0  calMaxX=Inf  calMinX=-Inf  calFormatX='-1'  calUnitX='Nm'  calHelpX=''  calAccess=1  calFunction=raptor_xcp_function(gcb)  measureEnable=off  mName=['Data1D_Output']
      settings: SourceProductName=Raptor
  Lim150 : Raptor_lib/Table Lookup/raptor_table_1d  dataName='CTRL_ThrottleToTorqueCmd150_1D'  initValue=[0;8;17;25;33;40;48;55;62;68;74;79;84;88;92;95;97;99;100;100;100]  dataType=single  storage=Calibration  initValueX=[0;5;10;15;20;25;30;35;40;45;50;55;60;65;70;75;80;85;90;95;100]  dataTypeXY=single  storageXY=Calibration  calVisible=on  showTable=on  calGain=1.0  calOffset=0.0  calMax=Inf  calMin=-Inf  calFormat='-1'  calUnit='pct'  calHelp=''  showBreakpoint=on  dataNameX=[]  calGainX=1.0  calOffsetX=0.0  calMaxX=Inf  calMinX=-Inf  calFormatX='-1'  calUnitX='Nm'  calHelpX=''  calAccess=1  calFunction=raptor_xcp_function(gcb)  measureEnable=off  mName=['Data1D_Output']
      settings: SourceProductName=Raptor
  Matt : Raptor_lib/Table Lookup/raptor_table_1d  dataName='CTRL_ThrottleToTorqueCmdMatt_1D'  initValue=[0;3;6;9;12;15;25;35;45;55;65;75;85;95;105;115;135;155;175;195;200]  dataType=single  storage=Calibration  initValueX=[0;5;10;15;20;25;30;35;40;45;50;55;60;65;70;75;80;85;90;95;100]  dataTypeXY=single  storageXY=Calibration  calVisible=on  showTable=on  calGain=1.0  calOffset=0.0  calMax=Inf  calMin=-Inf  calFormat='-1'  calUnit='pct'  calHelp=''  showBreakpoint=on  dataNameX=[]  calGainX=1.0  calOffsetX=0.0  calMaxX=Inf  calMinX=-Inf  calFormatX='-1'  calUnitX='Nm'  calHelpX=''  calAccess=1  calFunction=raptor_xcp_function(gcb)  measureEnable=off  mName=['Data1D_Output']
      settings: SourceProductName=Raptor
  Multiport Switch : MultiPortSwitch  Inputs=7  SaturateOnIntegerOverflow=off  InputSameDT=off
  Noah : Raptor_lib/Table Lookup/raptor_table_1d  dataName='CTRL_ThrottleToTorqueCmdNoah_1D'  initValue=[0;3;6;9;12;15;25;35;45;55;65;75;85;95;105;115;135;155;175;195;200]  dataType=single  storage=Calibration  initValueX=[0;5;10;15;20;25;30;35;40;45;50;55;60;65;70;75;80;85;90;95;100]  dataTypeXY=single  storageXY=Calibration  calVisible=on  showTable=on  calGain=1.0  calOffset=0.0  calMax=Inf  calMin=-Inf  calFormat='-1'  calUnit='pct'  calHelp=''  showBreakpoint=on  dataNameX=[]  calGainX=1.0  calOffsetX=0.0  calMaxX=Inf  calMinX=-Inf  calFormatX='-1'  calUnitX='Nm'  calHelpX=''  calAccess=1  calFunction=raptor_xcp_function(gcb)  measureEnable=off  mName=['Data1D_Output']
      settings: SourceProductName=Raptor
  Torque : Outport
  wires:
  Data Type Conversion/1 -> Add/1
  Constant/1 -> Add/2
  Add/1 -> Multiport Switch/1
  CTRL_TorqueCurve_en/1 -> Data Type Conversion/1
  Multiport Switch/1 -> Torque/1
  Lim100/1 -> Multiport Switch/8
  Lim150/1 -> Multiport Switch/7
  Carter/1 -> Multiport Switch/6
  Noah/1 -> Multiport Switch/5
  Casey/1 -> Multiport Switch/4
  Matt/1 -> Multiport Switch/3
  Default/1 -> Multiport Switch/2
  CTRL_ThrottlePosition_pct/1 -> Default/1, Matt/1, Casey/1, Noah/1, Carter/1, Lim100/1, Lim150/1  "100Nm Limit"

== matlab function TorqueCommand/ShifterState/MATLAB Function ==
  data: IO_PwrUpSwitch_bool input; IO_PwrDownSwitch_bool input; stateNum output
function stateNum = fcn(IO_PwrUpSwitch_bool, IO_PwrDownSwitch_bool)
 
persistent state prevUp prevDown
 
if isempty(state)

    state = TorqueState.State5;

end

if isempty(prevUp)

    prevUp = false;

    prevDown = false;

end
 
upButton = logical(IO_PwrUpSwitch_bool);

downButton = logical(IO_PwrDownSwitch_bool);
 
upEdge = (upButton && ~prevUp);

downEdge = (downButton && ~prevDown);
 
if upEdge

    newValue = min(uint8(state) + 1, 5);

    state = TorqueState(newValue);

elseif downEdge

    newValue = max(uint8(state) - 1, 0);

    state = TorqueState(newValue);

end
 
stateNum = uint8(state);
 
prevUp = upButton;

prevDown = downButton;

== stateflow chart TorqueCommand/TorqueProfiles/Chart ==
  state VehicleStatic
    state Default
      entry:
      Profile = TorqueProfile.Default;
      Curve = TorqueCurve.Default;
      TC = TCEnable.Off;
      Regen = RegenEnable.Off;
      Sensitivity = 5;
    state Testing2
      entry:
      Profile = TorqueProfile.Testing2;
      Curve = TorqueCurve.Lim100;
      TC = TCEnable.On;
      Regen = RegenEnable.On;
      Sensitivity = 5;
    state Driver1
      entry:
      Profile = TorqueProfile.Driver1;
      Curve = TorqueCurve.Matt;
      TC = TCEnable.On;
      Regen = RegenEnable.On;
      Sensitivity = 5;
    state Testing3
      entry:
      Profile = TorqueProfile.Testing3;
      Curve = TorqueCurve.Default;
      TC = TCEnable.On;
      Regen = RegenEnable.On;
      Sensitivity = 0;
    state Driver2
      entry:
      Profile = TorqueProfile.Driver2;
      Curve = TorqueCurve.Casey;
      TC = TCEnable.On;
      Regen = RegenEnable.On;
      Sensitivity = 5;
    state Testing4
      entry:
      Profile = TorqueProfile.Testing4;
      Curve = TorqueCurve.Default;
      TC = TCEnable.On;
      Regen = RegenEnable.On;
      Sensitivity = 1;
    state Driver3
      entry:
      Profile = TorqueProfile.Driver3;
      Curve = TorqueCurve.Noah;
      TC = TCEnable.On;
      Regen = RegenEnable.On;
      Sensitivity = 5;
    state Testing5
      entry:
      Profile = TorqueProfile.Testing5;
      Curve = TorqueCurve.Default;
      TC = TCEnable.On;
      Regen = RegenEnable.On;
      Sensitivity = 2;
    state Driver4
      entry:
      Profile = TorqueProfile.Driver4;
      Curve = TorqueCurve.Carter;
      TC = TCEnable.On;
      Regen = RegenEnable.On;
      Sensitivity = 5;
    state Testing6
      entry:
      Profile = TorqueProfile.Testing6;
      Curve = TorqueCurve.Default;
      TC = TCEnable.On;
      Regen = RegenEnable.On;
      Sensitivity = 3;
    state Testing1
      entry:
      Profile = TorqueProfile.Testing1;
      Curve = TorqueCurve.Lim150;
      TC = TCEnable.On;
      Regen = RegenEnable.On;
      Sensitivity = 5;
    (default) -> Default
    (junction 264) -> Default : [TCDial == 0]
    Testing2 -> (junction 276) : [TCDial ~= 6]
    (junction 47) -> (junction 264) [order 1]
    (junction 276) -> (junction 47)
    Default -> (junction 287) : [TCDial ~= 0]
    (junction 289) -> Testing2 : [TCDial == 6]
    (junction 287) -> (junction 47)
    (junction 47) -> (junction 289) [order 7]
    (junction 282) -> Driver1 : [TCDial == 1]
    Testing3 -> (junction 284) : [TCDial ~= 7]
    (junction 47) -> (junction 282) [order 2]
    (junction 284) -> (junction 47)
    Driver1 -> (junction 283) : [TCDial ~= 1]
    (junction 285) -> Testing3 : [TCDial == 7]
    (junction 283) -> (junction 47)
    (junction 47) -> (junction 285) [order 8]
    Testing4 -> (junction 269) : [TCDial ~= 8]
    (junction 273) -> Driver2 : [TCDial == 2]
    (junction 47) -> (junction 273) [order 3]
    (junction 269) -> (junction 47)
    (junction 274) -> (junction 47)
    (junction 47) -> (junction 267) [order 9]
    (junction 267) -> Testing4 : [TCDial == 8]
    (junction 47) -> (junction 271) [order 4]
    (junction 277) -> (junction 47)
    Driver2 -> (junction 274) : [TCDial ~= 2]
    (junction 272) -> (junction 47)
    (junction 47) -> (junction 278) [order 10]
    (junction 47) -> (junction 270) [order 5]
    (junction 280) -> (junction 47)
    (junction 268) -> (junction 47)
    (junction 47) -> (junction 279) [order 11]
    (junction 47) -> (junction 263) [order 6] : [TCDial == 5]
    (junction 281) -> (junction 47) : [TCDial ~= 5]
    (junction 271) -> Driver3 : [TCDial == 3]
    Testing5 -> (junction 277) : [TCDial ~= 9]
    Driver3 -> (junction 272) : [TCDial ~= 3]
    (junction 278) -> Testing5 : [TCDial == 9]
    (junction 270) -> Driver4 : [TCDial == 4]
    Testing6 -> (junction 280) : [TCDial ~= 10]
    Driver4 -> (junction 268) : [TCDial ~= 4]
    (junction 279) -> Testing6 : [TCDial == 10]
    (junction 263) -> Testing1
    Testing1 -> (junction 281)
  state ReadyToMove
    state NoTC
      entry:
      Sensitivity = 1;
    state Sens6
      entry:
      Sensitivity = 6;
    state Sens7
      entry:
      Sensitivity = 7;
    state Sens1
      entry:
      Sensitivity = 2;
    state Sens2
      entry:
      Sensitivity = 2;
    state Sens8
      entry:
      Sensitivity = 8;
    state Sens3
      entry:
      Sensitivity = 3;
    state Sens9
      entry:
      Sensitivity = 9;
    state Sens4
      entry:
      Sensitivity = 4;
    state Sens10
      entry:
      Sensitivity = 10;
    state Sens5
      entry:
      Sensitivity = 5;
    (default) -> NoTC
    (junction 395) -> NoTC : [TCDial == 0]
    Sens6 -> (junction 391) : [TCDial ~= 6]
    (junction 403) -> (junction 395) [order 1]
    (junction 391) -> (junction 403)
    NoTC -> (junction 396) : [TCDial ~= 0]
    (junction 397) -> Sens6 : [TCDial == 6]
    (junction 396) -> (junction 403)
    (junction 403) -> (junction 397) [order 7]
    (junction 390) -> Sens1 : [TCDial == 1]
    Sens7 -> (junction 392) : [TCDial ~= 7]
    (junction 403) -> (junction 390) [order 2]
    (junction 392) -> (junction 403)
    Sens1 -> (junction 394) : [TCDial ~= 1]
    (junction 393) -> Sens7 : [TCDial == 7]
    (junction 394) -> (junction 403)
    (junction 403) -> (junction 393) [order 8]
    Sens8 -> (junction 398) : [TCDial ~= 8]
    (junction 402) -> Sens2 : [TCDial == 2]
    (junction 403) -> (junction 402) [order 3]
    (junction 398) -> (junction 403)
    (junction 399) -> (junction 403)
    (junction 403) -> (junction 407) [order 9]
    (junction 407) -> Sens8 : [TCDial == 8]
    (junction 403) -> (junction 400) [order 4]
    (junction 401) -> (junction 403)
    Sens2 -> (junction 399) : [TCDial ~= 2]
    (junction 404) -> (junction 403)
    (junction 403) -> (junction 405) [order 10]
    (junction 403) -> (junction 406) [order 5]
    (junction 408) -> (junction 403)
    (junction 409) -> (junction 403)
    (junction 403) -> (junction 413) [order 11]
    (junction 403) -> (junction 410) [order 6]
    (junction 411) -> (junction 403)
    (junction 400) -> Sens3 : [TCDial == 3]
    Sens9 -> (junction 401) : [TCDial ~= 9]
    Sens3 -> (junction 404) : [TCDial ~= 3]
    (junction 405) -> Sens9 : [TCDial == 9]
    (junction 406) -> Sens4 : [TCDial == 4]
    Sens10 -> (junction 408) : [TCDial ~= 10]
    Sens4 -> (junction 409) : [TCDial ~= 4]
    (junction 413) -> Sens10 : [TCDial == 10]
    (junction 410) -> Sens5 : [TCDial == 5]
    Sens5 -> (junction 411) : [TCDial ~= 5]
  (default) -> VehicleStatic
  VehicleStatic -> ReadyToMove : [[State == VehicleState.ReadyToMove]]
  ReadyToMove -> VehicleStatic : [State ~= VehicleState.ReadyToMove]
  data: Profile output; Curve output; Sensitivity output; TCDial input; State input; Regen output; TC output
